simulink model "Simplus_1OL_2GFL"  (R2022b)
settings: Solver=ode3  StartTime=0.0  StopTime=35  FixedStep=Ts  RelTol=1e-3  EnableMultiTasking=on
InitFcn:
  | Ts = 100e-6;
model workspace (MAT data in the model file):
  Fbase = 50
  Filter_Ind = 0.00435
  Test_Interval = 5
  VDCref = 48
undefined symbols (not defined in the file): DiscIntNeverNeededParam
libraries: rtpi x45, spsabctodq0Lib x2, slpidlib x1, spsdq0toabcLib x1, simulink x1
settings Model: ModifiedByFormat=The MathWorks Inc.  SimulationMode=external  ExtModeTrigDuration=350000  ExtModeLogAll=off  Creator=The MathWorks, Inc.  LastModifiedBy=The MathWorks Inc.
settings SolverCC: AlgebraicLoopSolver=TrustRegion  PositivePriorityOrder=on  AutoInsertRateTranBlk=on
settings DataIOCC: LimitDataPoints=on  SaveFormat=Array  ReturnWorkspaceOutputs=off
settings OptimizationCC: EnhancedBackFolding=on  PassReuseOutputArgsThreshold=0  LocalBlockOutputs=off  EfficientMapNaN2IntZero=off  MaxStackSize=64  OptimizeBlockOrder=speed  DifferentSizesBufferReuse=on
settings DebuggingCC: UnderspecifiedInitializationDetection=Classic  MergeDetectMultiDrivingBlocksExec=none  SolverPrmCheckMsg=warning  ParameterTunabilityLossMsg=error  UnconnectedInputMsg=warning  UnconnectedOutputMsg=warning  UnconnectedLineMsg=warning  AllowSymbolicDim=off  SFUnexpectedBacktrackingDiag=warning  SFNoUnconditionalDefaultTransitionDiag=warning  SFExecutionAtInitializationDiag=none  SFMachineParentedDataDiag=warning  ArithmeticOperatorsInVariantConditions=warning
settings HardwareCC: ProdBitPerPointer=32  ProdBitPerSizeT=32  ProdBitPerPtrDiffT=32  ProdLargestAtomicInteger=Long  ProdLargestAtomicFloat=Double  ProdWordSize=32  ProdHWDeviceType=ARM Compatible->ARM Cortex  UseEmbeddedCoderFeatures=off
settings ModelReferenceCC: EnableRefExpFcnMdlSchedulingChecks=on  PropagateSignalLabelsOutOfModel=off
settings SFSimCC: SimUseLocalCustomCode=off  SimParseCustomCode=off  MATLABDynamicMemAlloc=off  CustomCodeUndefinedFunction=UseInterfaceOnly
settings RTWCC: Description=Simplus  SystemTargetFile=simplus.tlc  TemplateMakefile=simplex.tmf  RTWUseLocalCustomCode=off  RTWUseSimCustomCode=on  Toolchain=Simplus Xenomai ARM32  BuildConfiguration=Faster Runs
settings CodeAppCC: OperatorAnnotations=on  MangleLength=10  StateflowObjectComments=on
settings STFCustomTargetCC: TargetLangStandard=C99 (ISO)  GenerateFullHeader=off  ConcurrentExecutionCompliant=on  GRTInterface=on  UseToolchainInfoCompliant=on  SystemTargetFile=simplus.tlc
settings GRTTargetCC: GenerateFullHeader=off  ParMdlRefBuildCompliant=off  CompOptLevelCompliant=off  CombineOutputUpdateFcns=off  MatFileLogging=off  CPPClassGenCompliant=off  GRTInterface=on  ExtMode=on  ExtModeMexArgs='192.168.10.109', 0, 17725
settings ConfigComp: CovMetricSettings=dw  CovSaveCumulativeToWorkspaceVar=on  CovSaveSingleToWorkspaceVar=on  CovExternalEMLEnable=off  CovSFcnEnable=off

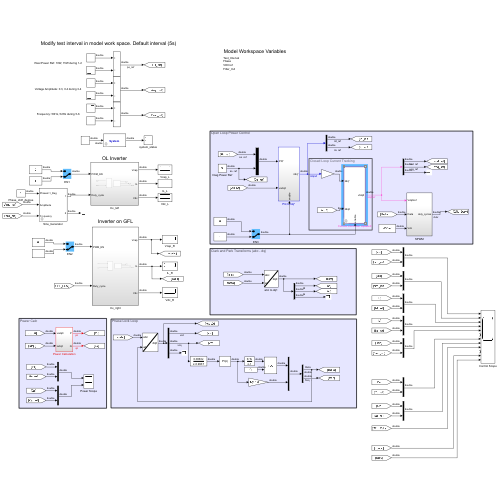
[thumbnail: Simulink's stored preview of the top-level diagram]
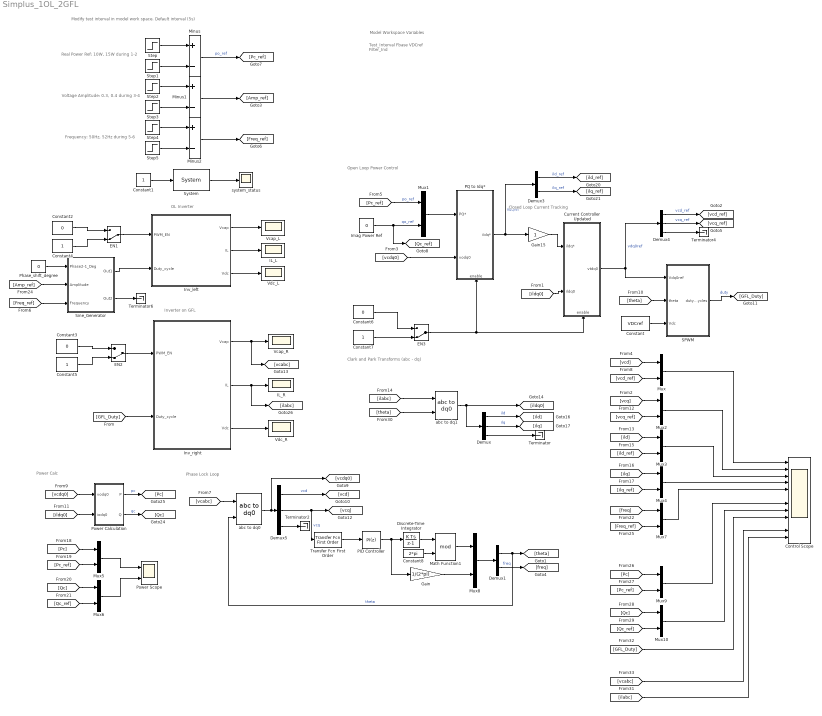
== system Simplus_1OL_2GFL ==
  note: Real Power Ref: 10W, 15W during 1-2
  note: Clark and Park Transforms (abc - dq)
  note: Closed Loop Current Tracking
  note: Phase Lock Loop
  note: Inverter on GFL
  note: Power Calc
  note: Open Loop Power Control
  note: OL Inverter
  note: Modify test interval in model work space. Default interval (5s)
  note: Voltage Amplitude: 0.3, 0.4 during 3-4
  note: Frequency: 50Hz, 52Hz during 5-6
  note: Test_Interval
      | Fbase
      | VDCref
      | Filter_Ind
  note: Model Workspace Variables
  Constant : Constant  Value=VDCref
  Constant{1,4..5,7} (4 alike) : Constant
  Constant2 : Constant  Value=0
  Constant3 : Constant  Value=0
  Constant6 : Constant  Value=0
  Constant8 : Constant  Value=2*pi
  Control Scope : Scope  NumInputPorts=12
  Current Controller Updated : Subsystem  mask{Id_Proportional=1.22, Id_Integral=957}
      mask prompts: Id_Proportional "Kp"; Id_Integral "Ki"
      settings: PortSchema="{\"entries\":[{\"content\":{\"sides\":[{\"content\":{\"connectorIds\":[\"In1\",\"In2\"]},\"type\":\"ConnectorPlacement.EquallySpacedRectSide\",\"uuid\":\"134caf41-c34b-48d0-a71a-522329c40d8c\"},{\"content\":{\"connectorIds\":[\"Out1\"],\"side\":\"RIGHT\"},\"type\":\"ConnectorPlacement.EquallySpacedRectSide\",\"uuid\":\"de6d8359-09d9-4cb7-8990-bc4b6d48f18d\"},{\"content\":{\"connectorIds\":[],\"side\":\"TOP\"},\"type\":\"ConnectorPlacement.EquallySpacedRectSide\",\"uuid\":\"e2785d07-2ead-4d42-94ac-8025f550e46a\"},{\"content\":{\"connectorIds\":[\"In3\"],\"side\":\"BOTTOM\"},\"type\":\"ConnectorPlacement.EquallySpacedRectSide\",\"uuid\":\"a912a274-012c-4cba-911c-beb79bb7dc91\"}]},\"type\":\"ConnectorPlacement.EquallySpacedConnector\",\"uuid\":\"3c498838-bb9a-4b09-bf48-00f71cabf7b4\"}],\"packageUris\":[\"http://schema.mathworks.com/mf0/Connector/R2020b\"],\"version\":\"1.0\"}"
  Demux : Demux  Outputs=3
  Demux1 : Demux  Outputs=2
  Demux3 : Demux  Outputs=2
  Demux4 : Demux  Outputs=3
  Demux5 : Demux  Outputs=3
  Discrete-Time Integrator : DiscreteIntegrator  SampleTime=Ts  ICPrevOutput=DiscIntNeverNeededParam  ICPrevScaledInput=DiscIntNeverNeededParam
  EN1 : ManualSwitch  CurrentSetting=0
  EN2 : ManualSwitch  CurrentSetting=0
  EN3 : ManualSwitch  CurrentSetting=0
  Gain : Gain  Gain=1/(2*pi)
  Gain15 : Gain
  IL_L : Scope
  IL_R : Scope
  Imag Power Ref : Constant  Value=0
  Inv_left : Subsystem
  Inv_right : Subsystem
  Math Function1 : Math  Operator=mod  SignedPower=on
  Minus : Sum  Inputs=+-
  Minus1 : Sum  Inputs=+-
  Minus2 : Sum  Inputs=+-
  Mux{,1..10} (11 alike) : Mux  Inputs=2
  PID Controller : slpidlib/PID Controller  Controller=PI  Form=Parallel  TimeDomain=Discrete-time  UseExternalTs=off  SampleTime=Ts  IntegratorMethod=Forward Euler  FilterMethod=Forward Euler  ControllerParametersSource=internal  P=2.4  I=1.52  UseKiTs=off  D=0  N=100  UseFilter=on  TunerSelectOption=Transfer Function Based (PID Tuner App)  InitialConditionSource=internal  InitialConditionForIntegrator=2*pi*Fbase  InitialConditionForFilter=0  DifferentiatorICPrevScaledInput=0  ExternalReset=none  TrackingMode=off  Kt=1  LimitOutput=off  SatLimitsSource=internal  UpperSaturationLimit=inf  LowerSaturationLimit=-inf  LinearizeAsGain=on  AntiWindupMode=none  Kb=1  LimitIntegrator=off  UpperIntegratorSaturationLimit=inf  LowerIntegratorSaturationLimit=-inf  POutMin=[]  POutMax=[]  IOutMin=[]  IOutMax=[]  DOutMin=[]  DOutMax=[]  NOutMin=[]  NOutMax=[]  SumOutMin=[]  SumOutMax=[]  SaturationOutMin=[]  SaturationOutMax=[]  PParamMin=[]  PParamMax=[]  IParamMin=[]  IParamMax=[]  DParamMin=[]  DParamMax=[]  NParamMin=[]  NParamMax=[]  KbParamMin=[]  KbParamMax=[]  KtParamMin=[]  KtParamMax=[]  KbOutMin=[]  KbOutMax=[]  KtOutMin=[]  KtOutMax=[]  IntegratorOutMin=[]  IntegratorOutMax=[]  FilterOutMin=[]  FilterOutMax=[]  SumI1OutMin=[]  SumI1OutMax=[]  SumI2OutMin=[]  SumI2OutMax=[]  SumI3OutMin=[]  SumI3OutMax=[]  SumI4OutMin=[]  SumI4OutMax=[]  SumDOutMin=[]  SumDOutMax=[]  DifferentiatorOutMin=[]  DifferentiatorOutMax=[]  FilterDiffOutCoefMin=[]  FilterDiffOutCoefMax=[]  ReciprocalOutMin=[]  ReciprocalOutMax=[]  SumDenOutMin=[]  SumDenOutMax=[]  SumNumOutMin=[]  SumNumOutMax=[]  DivideOutMin=[]  DivideOutMax=[]  UdiffTsProdOutMin=[]  UdiffTsProdOutMax=[]  NTsProdOutMin=[]  NTsProdOutMax=[]  UintegralTsProdOutMin=[]  UintegralTsProdOutMax=[]  UngainTsProdOutMin=[]  UngainTsProdOutMax=[]  ClampingZeroOutDataTypeStr=Inherit: Inherit via back propagation  ClampingZeroOutMin=[]  ClampingZeroOutMax=[]  FilterDenConstantOutDataTypeStr=Inherit: Inherit via back propagation  FilterDenConstantOutMin=[]  FilterDenConstantOutMax=[]  PCopyOutDataTypeStr=Inherit: Inherit via back propagation  PCopyOutMin=[]  PCopyOutMax=[]  NCopyOutDataTypeStr=Inherit: Inherit via back propagation  NCopyOutMin=[]  NCopyOutMax=[]  IntegratorContinuousStateAttributes=''  IntegratorStateMustResolveToSignalObject=off  IntegratorRTWStateStorageClass=Auto  FilterContinuousStateAttributes=''  FilterStateMustResolveToSignalObject=off  FilterRTWStateStorageClass=Auto  ParallelPVariant=InternalParameters  IdealPVariant=Disabled  IVariant=InternalParameters  DVariant=Disabled  IntegratorVariant=Discrete  SatVariant=Disabled  AWVariant=Passthrough  PCopyVariant=Disabled  TRVariant=Disabled  FdbkBlocksVariant=Forward  IdealPFdbkVariant=Disabled  SatFdbkVariant=Disabled  DerivativeFilterVariant=Disabled  NVariant=Disabled  NCopyVariant=Disabled_SignalSpec  FilterICVariant=Disabled  IntegratorICVariant=InternalICs  ExternalResetVariant=Disabled  TRSumVariant=Passthrough  SumFdbkVariant=Disabled  SumVariant=Sum_PI  TsampFilterVariant=InternalTs  TsampNgainVariant=Passthrough  TsampIntegralVariant=Passthrough  ExternalSaturationOutDataTypeStr=Inherit: Same as second input
  PQ to Idq* : Subsystem
      settings: PortSchema="{\"entries\":[{\"content\":{\"sides\":[{\"content\":{\"connectorIds\":[\"In1\",\"In2\"]},\"type\":\"ConnectorPlacement.EquallySpacedRectSide\",\"uuid\":\"5271b3ed-46a4-4113-9b69-458d23b85fa2\"},{\"content\":{\"connectorIds\":[\"Out1\"],\"side\":\"RIGHT\"},\"type\":\"ConnectorPlacement.EquallySpacedRectSide\",\"uuid\":\"00fb532b-4b50-4607-a5c4-cd74a5a5fc42\"},{\"content\":{\"connectorIds\":[],\"side\":\"TOP\"},\"type\":\"ConnectorPlacement.EquallySpacedRectSide\",\"uuid\":\"05671b8e-b1fa-45d3-a4a8-1640aa1af326\"},{\"content\":{\"connectorIds\":[\"In3\"],\"side\":\"BOTTOM\"},\"type\":\"ConnectorPlacement.EquallySpacedRectSide\",\"uuid\":\"cfa1ca65-6f63-4245-906b-c8bf76b96ed3\"}]},\"type\":\"ConnectorPlacement.EquallySpacedConnector\",\"uuid\":\"bf062c94-390f-4409-83d1-f8a32d59f496\"}],\"packageUris\":[\"http://schema.mathworks.com/mf0/Connector/R2020b\"],\"version\":\"1.0\"}"
  Phase_shift_degree : Constant  Value=0
  Power Calculation : Subsystem
  Power Scope : Scope  NumInputPorts=2
  SPWM : Subsystem
  Sine_Generator : Subsystem
  Step : Step  Time=Test_Interval*1  Before=10  After=15
  Step1 : Step  Time=Test_Interval*2  After=5
  Step2 : Step  Time=Test_Interval*3  Before=0.3  After=0.4
  Step3 : Step  Time=Test_Interval*4  After=0.1
  Step4 : Step  Time=Test_Interval*5  Before=50  After=52  SampleTime=0
  Step5 : Step  Time=Test_Interval*6  After=2
  System : rtpi/System  Priority=-100  finger_print=015482637925  sync=Synchronous Series  div=4  estop=NONE
      settings: SourceProductName=Simplus Real-Time
  Terminator{,2,4,6} (4 alike) : Terminator
  Transfer Fcn First Order : simulink/Discrete/Transfer Fcn First Order  PoleZ=0.9937  ICPrevOutput=0.0  DoSatur=off
  Vcap_L : Scope
  Vcap_R : Scope
  Vdc_L : Scope
  Vdc_R : Scope
  abc to dq0 : spsabctodq0Lib/abc to dq0  Alignment=90 degrees behind phase A axis
  abc to dq1 : spsabctodq0Lib/abc to dq0  Alignment=90 degrees behind phase A axis
  system_status : Scope
  wires:
  System/1 -> system_status/1
  Constant1/1 -> System/1
  Constant2/1 -> EN1/1
  Constant4/1 -> EN1/2
  Constant5/1 -> EN2/2
  Constant3/1 -> EN2/1
  Inv_left/1(Vcap) -> Vcap_L/1
  EN1/1 -> Inv_left/1(PWM_EN)
  Sine_Generator/1(Out1) -> Inv_left/2(Duty_cycle)
  Inv_left/2(IL) -> IL_L/1
  Inv_left/3(Vdc) -> Vdc_L/1
  Inv_right/1(Vcap) -> [vcabc], Vcap_R/1
  EN2/1 -> Inv_right/1(PWM_EN)
  Inv_right/2(IL) -> [ilabc], IL_R/1
  Inv_right/3(Vdc) -> Vdc_R/1
  Phase_shift_degree/1 -> Sine_Generator/1(Phase2-1_Deg)
  Demux4/2 -> [vcq_ref]  "vcq_ref"
  Demux/2 -> [ilq]  "ilq"
  Demux4/3 -> Terminator4/1
  Demux3/2 -> [ilq_ref]  "ilq_ref"
  Demux/3 -> Terminator/1
  PQ to Idq*/1(iIdq*) -> Gain15/1, Demux3/1  "ildqref"
  Current Controller Updated/1(vtdq0) -> SPWM/1(Vdq0ref), Demux4/1  "vdq0ref"
  [theta] -> SPWM/2(theta)
  SPWM/1(duty_cycles) -> [GFL_Duty]  "duty"
  Power Calculation/2(Q) -> [Qc]  "qc"
  Demux/1 -> [ild]  "ild"
  EN3/1 -> Current Controller Updated/3(enable), PQ to Idq*/3(enable)
  Power Calculation/1(P) -> [Pc]  "pc"
  Demux3/1 -> [ild_ref]  "ild_ref"
  [ildq0] -> Power Calculation/2(iodq0)
  Demux4/1 -> [vcd_ref]  "vcd_ref"
  [vcdq0] -> Power Calculation/1(vodq0)
  Constant/1 -> SPWM/3(Vdc)
  Gain15/1 -> Current Controller Updated/1(ildq*)
  Sine_Generator/2(Out2) -> Terminator6/1
  [GFL_Duty] -> Inv_right/2(Duty_cycle)
  Constant6/1 -> EN3/1
  Constant7/1 -> EN3/2
  [vcd_ref] -> Mux/2
  [vcd] -> Mux/1
  [vcq] -> Mux2/1
  [vcq_ref] -> Mux2/2
  [ild] -> Mux3/1
  [ild_ref] -> Mux3/2
  [ilq] -> Mux4/1
  [ilq_ref] -> Mux4/2
  Mux/1 -> Control Scope/1
  Mux2/1 -> Control Scope/2
  Mux3/1 -> Control Scope/3
  Mux4/1 -> Control Scope/4
  PID Controller/1 -> Gain/1, Discrete-Time Integrator/1
  Gain/1 -> Mux8/2
  Discrete-Time Integrator/1 -> Math Function1/1
  Constant8/1 -> Math Function1/2
  Demux1/2 -> [freq]  "freq"
  Demux1/1 -> abc to dq0/2, [theta]  "theta"
  Mux8/1 -> Demux1/1
  abc to dq0/1 -> [vcdq0], Demux5/1
  Demux5/1 -> [vcd]  "vcd"
  Demux5/3 -> Terminator2/1
  Demux5/2 -> Transfer Fcn First Order/1, [vcq]  "vcq"
  [vcabc] -> abc to dq0/1
  [theta] -> abc to dq1/2
  abc to dq1/1 -> [ildq0], Demux/1
  Mux6/1 -> Power Scope/2
  [Pc_ref] -> Mux5/2
  [Pc] -> Mux5/1
  [Qc_ref] -> Mux6/2
  [Qc] -> Mux6/1
  Mux5/1 -> Power Scope/1
  [Pc] -> Mux9/1
  [Qc] -> Mux10/1
  [Pc_ref] -> Mux9/2
  [Qc_ref] -> Mux10/2
  [ilabc] -> Control Scope/12
  Mux9/1 -> Control Scope/7
  [vcabc] -> Control Scope/11
  Mux10/1 -> Control Scope/8
  [GFL_Duty] -> Control Scope/9
  Mux1/1 -> PQ to Idq*/1(PQ*)
  Imag Power Ref/1 -> [Qc_ref], Mux1/2  "qo_ref"
  [Pc_ref] -> Mux1/1  "po_ref"
  [vcdq0] -> PQ to Idq*/2(vodq0)
  [ildq0] -> Current Controller Updated/2(ildq0)
  [ilabc] -> abc to dq1/1
  Step/1 -> Minus/1
  Step1/1 -> Minus/2
  Step2/1 -> Minus1/1
  Step3/1 -> Minus1/2
  Step4/1 -> Minus2/1
  Step5/1 -> Minus2/2
  Minus/1 -> [Pc_ref]  "po_ref"
  Minus1/1 -> [Amp_ref]
  Minus2/1 -> [Freq_ref]
  [Amp_ref] -> Sine_Generator/2(Amplitude)
  [Freq_ref] -> Sine_Generator/3(Frequency)
  [Freq_ref] -> Mux7/2
  [freq] -> Mux7/1
  Mux7/1 -> Control Scope/5
  Math Function1/1 -> Mux8/1
  Transfer Fcn First Order/1 -> PID Controller/1

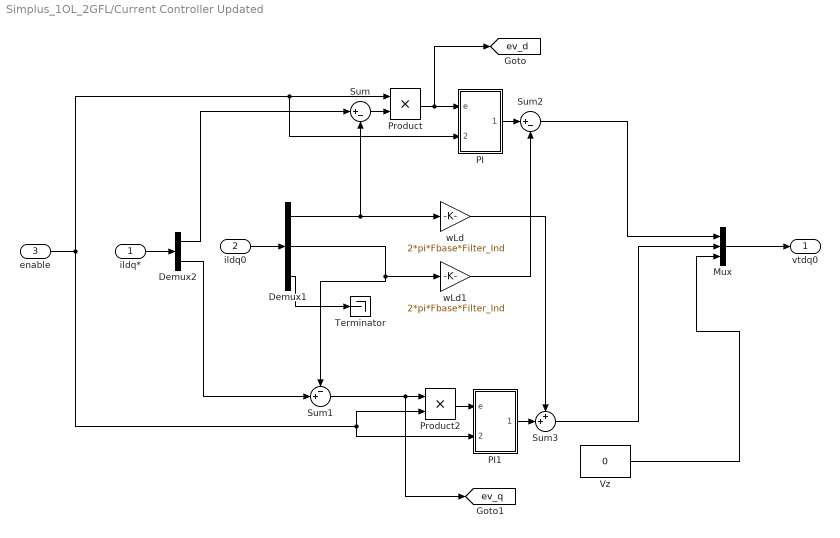
== system Simplus_1OL_2GFL/Current Controller Updated ==
  ildq* : Inport
  ildq0 : Inport  Port=2
  enable : Inport  Port=3
  Demux1 : Demux  Outputs=3
  Demux2 : Demux  Outputs=2
  Mux : Mux  Inputs=3
  PI : Subsystem
  PI1 : Subsystem
  Product : Product  RndMeth=Zero
  Product2 : Product  RndMeth=Zero
  Sum : Sum  Inputs=|+-
  Sum1 : Sum  Inputs=-+|
  Sum2 : Sum  Inputs=|+-
  Sum3 : Sum  Inputs=++|
  Terminator : Terminator
  Vz : Constant  Value=0
  wLd : Gain  Gain=2*pi*Fbase*Filter_Ind
  wLd1 : Gain  Gain=2*pi*Fbase*Filter_Ind
  vtdq0 : Outport
  tag scope: ev_d=global, ev_q=global
  wires:
  Sum2/1 -> Mux/1
  Sum3/1 -> Mux/2
  ildq0/1 -> Demux1/1
  Mux/1 -> vtdq0/1
  Demux1/3 -> Terminator/1
  ildq*/1 -> Demux2/1
  Demux2/1 -> Sum/1
  Demux2/2 -> Sum1/2
  Product/1 -> [ev_d], PI/1(e)
  Sum1/1 -> [ev_q], Product2/1
  PI/1(Out) -> Sum2/1
  wLd/1 -> Sum3/1
  wLd1/1 -> Sum2/2
  PI1/1(Out) -> Sum3/2
  Demux1/2 -> Sum1/1, wLd1/1
  Demux1/1 -> wLd/1, Sum/2
  Product2/1 -> PI1/1(e)
  Sum/1 -> Product/2
  enable/1 -> Product/1, PI/2(RST), PI1/2(RST), Product2/2
  Vz/1 -> Mux/3

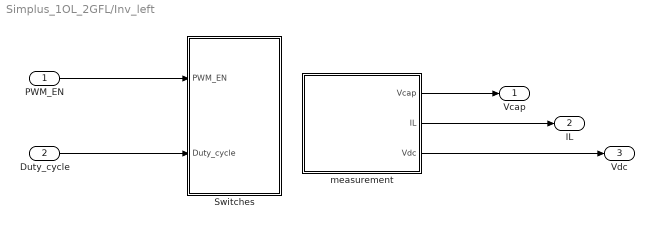
== system Simplus_1OL_2GFL/Inv_left ==
  PWM_EN : Inport
  Duty_cycle : Inport  Port=2
  Switches : Subsystem
  measurement : Subsystem
  Vcap : Outport
  IL : Outport  Port=2
  Vdc : Outport  Port=3
  wires:
  Duty_cycle/1 -> Switches/2(Duty_cycle)
  PWM_EN/1 -> Switches/1(PWM_EN)
  measurement/3(Vdc) -> Vdc/1
  measurement/2(IL) -> IL/1
  measurement/1(Vcap) -> Vcap/1

== system Simplus_1OL_2GFL/Inv_right ==
  PWM_EN : Inport
  Duty_cycle : Inport  Port=2
  Switches : Subsystem
  measurement : Subsystem
  Vcap : Outport
  IL : Outport  Port=2
  Vdc : Outport  Port=3
  wires:
  measurement/1(Vcap) -> Vcap/1
  measurement/2(IL) -> IL/1
  measurement/3(Vdc) -> Vdc/1
  PWM_EN/1 -> Switches/1(PWM_EN)
  Duty_cycle/1 -> Switches/2(Duty_cycle)

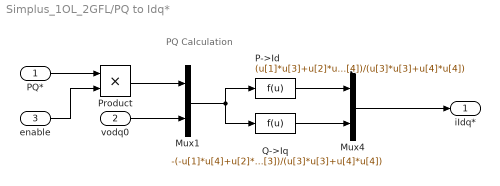
== system Simplus_1OL_2GFL/PQ to Idq* ==
  note: PQ Calculation
  PQ* : Inport
  vodq0 : Inport  Port=2
  enable : Inport  Port=3
  Mux1 : Mux  Inputs=2
  Mux4 : Mux  Inputs=2
  P->Id : Fcn  Expr=(u[1]*u[3]+u[2]*u[4])/(u[3]*u[3]+u[4]*u[4])
  Product : Product  RndMeth=Zero
  Q->Iq : Fcn  Expr=-(-u[1]*u[4]+u[2]*u[3])/(u[3]*u[3]+u[4]*u[4])
  iIdq* : Outport
  wires:
  enable/1 -> Product/2
  Product/1 -> Mux1/1
  Mux1/1 -> P->Id/1, Q->Iq/1
  P->Id/1 -> Mux4/1
  Q->Iq/1 -> Mux4/2
  Mux4/1 -> iIdq*/1
  vodq0/1 -> Mux1/2
  PQ*/1 -> Product/1

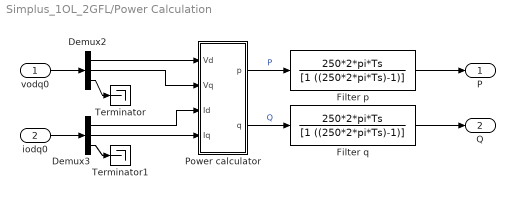
== system Simplus_1OL_2GFL/Power Calculation ==
  vodq0 : Inport
  iodq0 : Inport  Port=2
  Demux2 : Demux  Outputs=3
  Demux3 : Demux  Outputs=3
  Filter p : DiscreteTransferFcn  Numerator=250*2*pi*Ts  Denominator=[1 ((250*2*pi*Ts)-1)]  SampleTime=Ts
  Filter q : DiscreteTransferFcn  Numerator=250*2*pi*Ts  Denominator=[1 ((250*2*pi*Ts)-1)]  SampleTime=Ts
  Power calculator : Subsystem
  Terminator : Terminator
  Terminator1 : Terminator
  P : Outport
  Q : Outport  Port=2
  wires:
  vodq0/1 -> Demux2/1
  Demux2/1 -> Power calculator/1(Vd)
  Demux2/2 -> Power calculator/2(Vq)
  Demux3/1 -> Power calculator/3(Id)
  Demux3/2 -> Power calculator/4(Iq)
  iodq0/1 -> Demux3/1
  Power calculator/1(p) -> Filter p/1  "P"
  Power calculator/2(q) -> Filter q/1  "Q"
  Demux2/3 -> Terminator/1
  Demux3/3 -> Terminator1/1
  Filter p/1 -> P/1
  Filter q/1 -> Q/1

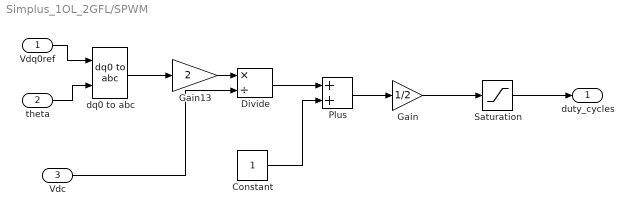
== system Simplus_1OL_2GFL/SPWM ==
  Vdq0ref : Inport
  theta : Inport  Port=2
  Vdc : Inport  Port=3
  Constant : Constant
  Divide : Product  Inputs=*/
  Gain : Gain  Gain=1/2
  Gain13 : Gain  Gain=2
  Plus : Sum
  Saturation : Saturate  UpperLimit=0.9  LowerLimit=0.1
  dq0 to abc : spsdq0toabcLib/dq0 to abc  Alignment=90 degrees behind phase A axis
  duty_cycles : Outport
  wires:
  Vdq0ref/1 -> dq0 to abc/1
  Gain/1 -> Saturation/1
  theta/1 -> dq0 to abc/2
  Constant/1 -> Plus/2
  Plus/1 -> Gain/1
  Saturation/1 -> duty_cycles/1
  dq0 to abc/1 -> Gain13/1
  Gain13/1 -> Divide/1
  Vdc/1 -> Divide/2
  Divide/1 -> Plus/1

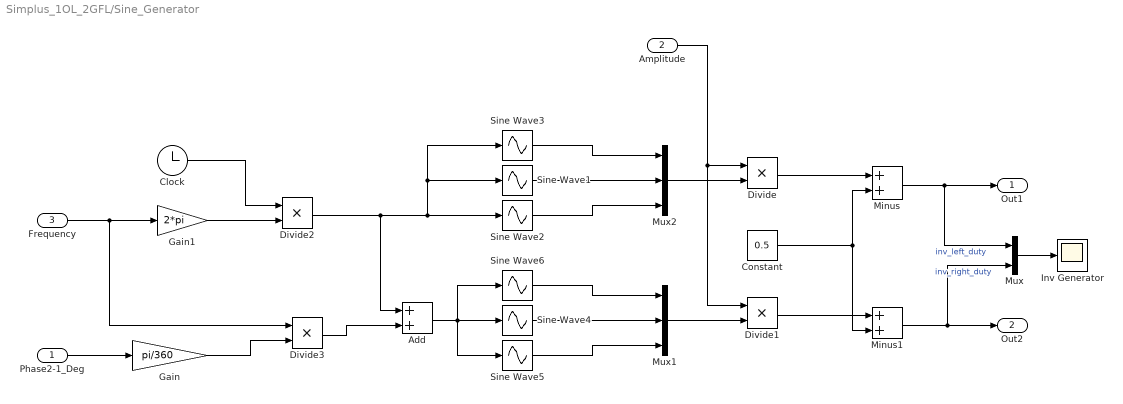
== system Simplus_1OL_2GFL/Sine_Generator ==
  Phase2-1_Deg : Inport
  Amplitude : Inport  Port=2
  Frequency : Inport  Port=3
  Add : Sum
  Clock : Clock
  Constant : Constant  Value=0.5
  Divide{,1..3} (4 alike) : Product  Inputs=**
  Gain : Gain  Gain=pi/360
  Gain1 : Gain  Gain=2*pi
  Inv Generator : Scope
  Minus : Sum
  Minus1 : Sum
  Mux : Mux  Inputs=2
  Mux1 : Mux  Inputs=3
  Mux2 : Mux  Inputs=3
  Sine Wave1 : Sin  TimeSource=Use external signal  Phase=-2*pi/3
  Sine Wave2 : Sin  TimeSource=Use external signal  Phase=2*pi/3
  Sine Wave3 : Sin  TimeSource=Use external signal
  Sine Wave4 : Sin  TimeSource=Use external signal  Phase=-2*pi/3
  Sine Wave5 : Sin  TimeSource=Use external signal  Phase=2*pi/3
  Sine Wave6 : Sin  TimeSource=Use external signal
  Out1 : Outport
  Out2 : Outport  Port=2
  wires:
  Add/1 -> Sine Wave6/1, Sine Wave5/1, Sine Wave4/1
  Sine Wave3/1 -> Mux2/1
  Divide2/1 -> Add/1, Sine Wave1/1, Sine Wave3/1, Sine Wave2/1
  Sine Wave6/1 -> Mux1/1
  Divide3/1 -> Add/2
  Sine Wave5/1 -> Mux1/3
  Sine Wave4/1 -> Mux1/2
  Sine Wave1/1 -> Mux2/2
  Sine Wave2/1 -> Mux2/3
  Minus/1 -> Out1/1, Mux/1  "inv_left_duty"
  Phase2-1_Deg/1 -> Gain/1
  Mux2/1 -> Divide/2
  Mux1/1 -> Divide1/2
  Amplitude/1 -> Divide/1, Divide1/1
  Gain1/1 -> Divide2/2
  Frequency/1 -> Divide3/1, Gain1/1
  Divide/1 -> Minus/1
  Divide1/1 -> Minus1/1
  Constant/1 -> Minus1/2, Minus/2
  Clock/1 -> Divide2/1
  Gain/1 -> Divide3/2
  Minus1/1 -> Out2/1, Mux/2  "inv_right_duty"
  Mux/1 -> Inv Generator/1

== system Simplus_1OL_2GFL/Current Controller Updated/PI ==
  e : Inport
  RST : Inport  Port=2
  Discrete-Time Integrator : DiscreteIntegrator  gainval=1  ExternalReset=either  SampleTime=Ts  LimitOutput=on  UpperSaturationLimit=20000  LowerSaturationLimit=-20000  ICPrevOutput=DiscIntNeverNeededParam  ICPrevScaledInput=DiscIntNeverNeededParam
  Ki : Gain  Gain=Id_Integral  SaturateOnIntegerOverflow=on  OutDataTypeStr=Inherit: Same as input  ParamDataTypeStr=Inherit: Same as input
  Kp : Gain  Gain=Id_Proportional  SaturateOnIntegerOverflow=on  OutDataTypeStr=Inherit: Same as input  ParamDataTypeStr=Inherit: Same as input
  Sum4 : Sum  SaturateOnIntegerOverflow=on
  Out : Outport
  wires:
  Ki/1 -> Discrete-Time Integrator/1
  Kp/1 -> Sum4/1
  e/1 -> Ki/1, Kp/1
  Discrete-Time Integrator/1 -> Sum4/2
  Sum4/1 -> Out/1
  RST/1 -> Discrete-Time Integrator/2

== system Simplus_1OL_2GFL/Current Controller Updated/PI1 ==
  e : Inport
  RST : Inport  Port=2
  Discrete-Time Integrator : DiscreteIntegrator  gainval=1  ExternalReset=either  SampleTime=Ts  LimitOutput=on  UpperSaturationLimit=20000  LowerSaturationLimit=-20000  ICPrevOutput=DiscIntNeverNeededParam  ICPrevScaledInput=DiscIntNeverNeededParam
  Ki : Gain  Gain=Id_Integral  SaturateOnIntegerOverflow=on  OutDataTypeStr=Inherit: Same as input  ParamDataTypeStr=Inherit: Same as input
  Kp : Gain  Gain=Id_Proportional  SaturateOnIntegerOverflow=on  OutDataTypeStr=Inherit: Same as input  ParamDataTypeStr=Inherit: Same as input
  Sum4 : Sum  SaturateOnIntegerOverflow=on
  Out : Outport
  wires:
  Ki/1 -> Discrete-Time Integrator/1
  Kp/1 -> Sum4/1
  e/1 -> Ki/1, Kp/1
  Discrete-Time Integrator/1 -> Sum4/2
  Sum4/1 -> Out/1
  RST/1 -> Discrete-Time Integrator/2

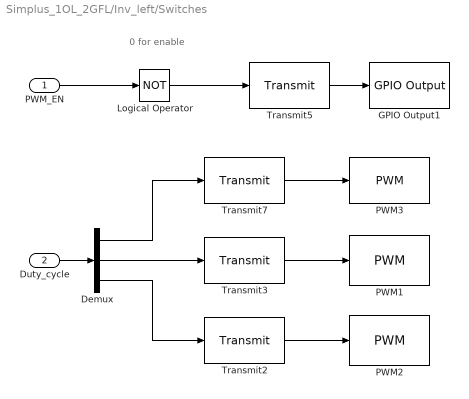
== system Simplus_1OL_2GFL/Inv_left/Switches ==
  note: 0 for enable
  PWM_EN : Inport
  Duty_cycle : Inport  Port=2
  Demux : Demux  Outputs=3
  GPIO Output1 : rtpi/GPIO Output  finger_print=115482637925  blk_num=1  gpio_num=1  gpio1=18  od1=off  gpio2=0  od2=off  gpio3=0  od3=off  gpio4=0  od4=off  gpio5=0  od5=off  gpio6=0  od6=off  gpio7=0  od7=off  gpio8=0  od8=off  gpio9=0  od9=off  gpio10=0  od10=off  gpio11=0  od11=off  gpio12=0  od12=off  gpio13=0  od13=off  gpio14=0  od14=off  gpio15=0  od15=off  gpio16=0  od16=off  dir=1
      settings: SourceProductName=Simplus Real-Time
  Logical Operator : Logic  Operator=NOT  AllPortsSameDT=off  OutDataTypeStr=boolean
  PWM1 : rtpi/PWM  finger_print=115482637925  blk_num=1  pwmx=5  sync=on  mode=Normal  input=Duty Cycle  data_type=float  trigger_a=Zero  trigger_b=Zero  clock=1  tdead=2  period=10000  duty=0.5  phase=0.0
      settings: SourceProductName=Simplus Real-Time
  PWM2 : rtpi/PWM  finger_print=115482637925  blk_num=2  pwmx=6  sync=on  mode=Normal  input=Duty Cycle  data_type=float  trigger_a=Zero  trigger_b=Zero  clock=1  tdead=2  period=10000  duty=0.5  phase=0.0
      settings: SourceProductName=Simplus Real-Time
  PWM3 : rtpi/PWM  finger_print=115482637925  blk_num=3  pwmx=4  sync=on  mode=Normal  input=Duty Cycle  data_type=float  trigger_a=Zero  trigger_b=Zero  clock=1  tdead=2  period=10000  duty=0.5  phase=0.0
      settings: SourceProductName=Simplus Real-Time
  Transmit2 : rtpi/Transmit  Priority=10  finger_print=115482637925  blk_num=1  data_type=4  conv_type=single
      settings: SourceProductName=Simplus Real-Time
  Transmit3 : rtpi/Transmit  Priority=10  finger_print=115482637925  blk_num=2  data_type=4  conv_type=single
      settings: SourceProductName=Simplus Real-Time
  Transmit5 : rtpi/Transmit  finger_print=115482637925  blk_num=3  data_type=2  conv_type=uint16
      settings: SourceProductName=Simplus Real-Time
  Transmit7 : rtpi/Transmit  Priority=10  finger_print=115482637925  blk_num=4  data_type=4  conv_type=single
      settings: SourceProductName=Simplus Real-Time
  wires:
  Transmit2/1 -> PWM2/1
  Transmit3/1 -> PWM1/1
  Transmit7/1 -> PWM3/1
  Duty_cycle/1 -> Demux/1
  Demux/2 -> Transmit3/1
  Demux/1 -> Transmit7/1
  Demux/3 -> Transmit2/1
  Transmit5/1 -> GPIO Output1/1
  Logical Operator/1 -> Transmit5/1
  PWM_EN/1 -> Logical Operator/1

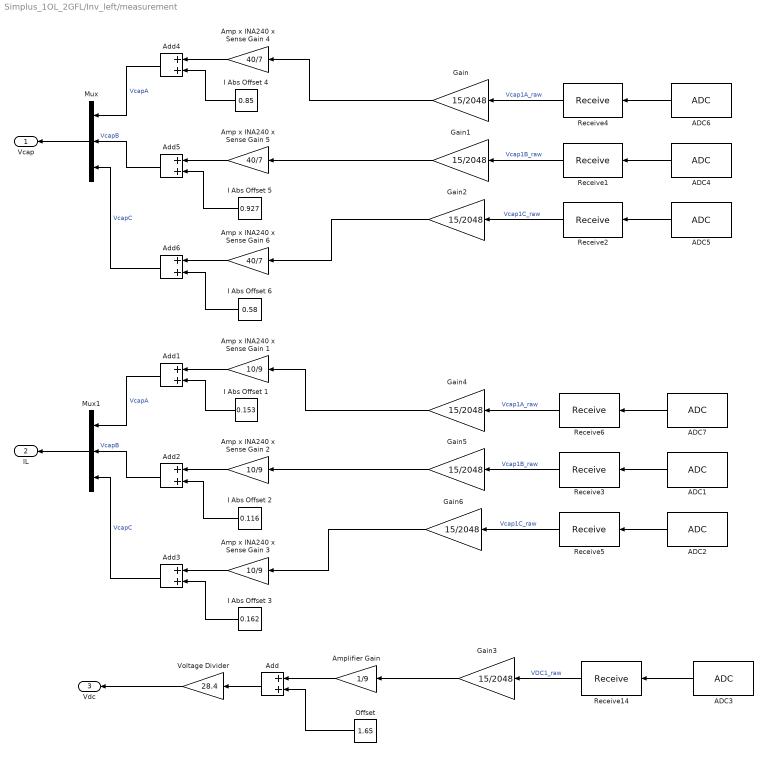
== system Simplus_1OL_2GFL/Inv_left/measurement ==
  ADC1 : rtpi/ADC  finger_print=115482637925  blk_num=1  adcx=D  prior=2  pin=D2  trigger=PWM4A  data_type=int16  gain=1  rsrc=100  offset=AC  protect=Enabled  max=1500  min=-1500
      settings: SourceProductName=Simplus Real-Time
  ADC2 : rtpi/ADC  finger_print=115482637925  blk_num=2  adcx=D  prior=3  pin=D3  trigger=PWM4A  data_type=int16  gain=1  rsrc=100  offset=AC  protect=Enabled  max=1500  min=-1500
      settings: SourceProductName=Simplus Real-Time
  ADC3 : rtpi/ADC  finger_print=115482637925  blk_num=3  adcx=D  prior=4  pin=D4  trigger=PWM4A  data_type=int16  gain=1  rsrc=100  offset=AC  protect=Enabled  max=1500  min=-2048
      settings: SourceProductName=Simplus Real-Time
  ADC4 : rtpi/ADC  finger_print=115482637925  blk_num=4  adcx=C  prior=2  pin=C2  trigger=PWM4A  data_type=int16  gain=1  rsrc=100  offset=AC  protect=Enabled  max=1500  min=-1500
      settings: SourceProductName=Simplus Real-Time
  ADC5 : rtpi/ADC  finger_print=115482637925  blk_num=5  adcx=C  prior=3  pin=C3  trigger=PWM4A  data_type=int16  gain=1  rsrc=100  offset=AC  protect=Enabled  max=1500  min=-1500
      settings: SourceProductName=Simplus Real-Time
  ADC6 : rtpi/ADC  finger_print=115482637925  blk_num=6  adcx=C  prior=1  pin=C1  trigger=PWM4A  data_type=int16  gain=1  rsrc=100  offset=AC  protect=Enabled  max=1500  min=-1500
      settings: SourceProductName=Simplus Real-Time
  ADC7 : rtpi/ADC  finger_print=115482637925  blk_num=7  adcx=D  prior=1  pin=D1  trigger=PWM4A  data_type=int16  gain=1  rsrc=100  offset=AC  protect=Enabled  max=1500  min=-1500
      settings: SourceProductName=Simplus Real-Time
  Add{,1..6} (7 alike) : Sum
  Amp x INA240 x Sense Gain 1 : Gain  Gain=10/9
  Amp x INA240 x Sense Gain 2 : Gain  Gain=10/9
  Amp x INA240 x Sense Gain 3 : Gain  Gain=10/9
  Amp x INA240 x Sense Gain 4 : Gain  Gain=40/7
  Amp x INA240 x Sense Gain 5 : Gain  Gain=40/7
  Amp x INA240 x Sense Gain 6 : Gain  Gain=40/7
  Amplifier Gain : Gain  Gain=1/9
  Gain{,1..6} (7 alike) : Gain  Gain=15/2048
  I Abs Offset 1 : Constant  Value=0.153
  I Abs Offset 2 : Constant  Value=0.116
  I Abs Offset 3 : Constant  Value=0.162
  I Abs Offset 4 : Constant  Value=0.85
  I Abs Offset 5 : Constant  Value=0.927
  I Abs Offset 6 : Constant  Value=0.58
  Mux : Mux  Inputs=3
  Mux1 : Mux  Inputs=3
  Offset : Constant  Value=1.65
  Receive1 : rtpi/Receive  Priority=12  finger_print=115482637925  blk_num=1  data_type=2
      settings: SourceProductName=Simplus Real-Time
  Receive14 : rtpi/Receive  Priority=12  finger_print=115482637925  blk_num=2  data_type=2
      settings: SourceProductName=Simplus Real-Time
  Receive2 : rtpi/Receive  Priority=12  finger_print=115482637925  blk_num=3  data_type=2
      settings: SourceProductName=Simplus Real-Time
  Receive3 : rtpi/Receive  Priority=12  finger_print=115482637925  blk_num=4  data_type=2
      settings: SourceProductName=Simplus Real-Time
  Receive4 : rtpi/Receive  Priority=12  finger_print=115482637925  blk_num=5  data_type=2
      settings: SourceProductName=Simplus Real-Time
  Receive5 : rtpi/Receive  Priority=12  finger_print=115482637925  blk_num=6  data_type=2
      settings: SourceProductName=Simplus Real-Time
  Receive6 : rtpi/Receive  Priority=12  finger_print=115482637925  blk_num=7  data_type=2
      settings: SourceProductName=Simplus Real-Time
  Voltage Divider : Gain  Gain=28.4
  Vcap : Outport
  IL : Outport  Port=2
  Vdc : Outport  Port=3
  wires:
  ADC6/1 -> Receive4/1
  Receive4/1 -> Gain/1  "Vcap1A_raw"
  Amp x INA240 x Sense Gain 6/1 -> Add6/1
  I Abs Offset 6/1 -> Add6/2
  I Abs Offset 4/1 -> Add4/2
  Amp x INA240 x Sense Gain 4/1 -> Add4/1
  ADC5/1 -> Receive2/1
  Amp x INA240 x Sense Gain 5/1 -> Add5/1
  Receive1/1 -> Gain1/1  "Vcap1B_raw"
  I Abs Offset 5/1 -> Add5/2
  Receive2/1 -> Gain2/1  "Vcap1C_raw"
  ADC4/1 -> Receive1/1
  Amp x INA240 x Sense Gain 3/1 -> Add3/1
  Amp x INA240 x Sense Gain 1/1 -> Add1/1
  I Abs Offset 1/1 -> Add1/2
  Amp x INA240 x Sense Gain 2/1 -> Add2/1
  I Abs Offset 2/1 -> Add2/2
  I Abs Offset 3/1 -> Add3/2
  Receive14/1 -> Gain3/1  "VDC1_raw"
  ADC3/1 -> Receive14/1
  Add/1 -> Voltage Divider/1
  Amplifier Gain/1 -> Add/1
  Offset/1 -> Add/2
  Voltage Divider/1 -> Vdc/1
  Gain/1 -> Amp x INA240 x Sense Gain 4/1
  Gain1/1 -> Amp x INA240 x Sense Gain 5/1
  Gain2/1 -> Amp x INA240 x Sense Gain 6/1
  Gain3/1 -> Amplifier Gain/1
  Add4/1 -> Mux/1  "VcapA"
  Add5/1 -> Mux/2  "VcapB"
  Add6/1 -> Mux/3  "VcapC"
  Mux/1 -> Vcap/1
  ADC7/1 -> Receive6/1
  Gain4/1 -> Amp x INA240 x Sense Gain 1/1
  Gain5/1 -> Amp x INA240 x Sense Gain 2/1
  ADC1/1 -> Receive3/1
  ADC2/1 -> Receive5/1
  Receive3/1 -> Gain5/1  "Vcap1B_raw"
  Receive5/1 -> Gain6/1  "Vcap1C_raw"
  Gain6/1 -> Amp x INA240 x Sense Gain 3/1
  Receive6/1 -> Gain4/1  "Vcap1A_raw"
  Add3/1 -> Mux1/3  "VcapC"
  Mux1/1 -> IL/1
  Add1/1 -> Mux1/1  "VcapA"
  Add2/1 -> Mux1/2  "VcapB"

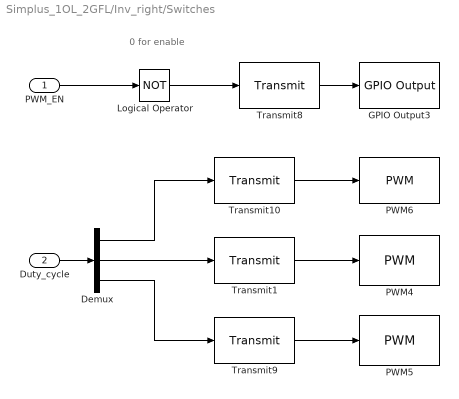
== system Simplus_1OL_2GFL/Inv_right/Switches ==
  note: 0 for enable
  PWM_EN : Inport
  Duty_cycle : Inport  Port=2
  Demux : Demux  Outputs=3
  GPIO Output3 : rtpi/GPIO Output  finger_print=115482637925  blk_num=2  gpio_num=1  gpio1=24  od1=off  gpio2=0  od2=off  gpio3=0  od3=off  gpio4=0  od4=off  gpio5=0  od5=off  gpio6=0  od6=off  gpio7=0  od7=off  gpio8=0  od8=off  gpio9=0  od9=off  gpio10=0  od10=off  gpio11=0  od11=off  gpio12=0  od12=off  gpio13=0  od13=off  gpio14=0  od14=off  gpio15=0  od15=off  gpio16=0  od16=off  dir=1
      settings: SourceProductName=Simplus Real-Time
  Logical Operator : Logic  Operator=NOT  AllPortsSameDT=off  OutDataTypeStr=boolean
  PWM4 : rtpi/PWM  finger_print=115482637925  blk_num=4  pwmx=2  sync=on  mode=Normal  input=Duty Cycle  data_type=float  trigger_a=Zero  trigger_b=Zero  clock=1  tdead=2  period=10000  duty=0.5  phase=0.0
      settings: SourceProductName=Simplus Real-Time
  PWM5 : rtpi/PWM  finger_print=115482637925  blk_num=5  pwmx=3  sync=on  mode=Normal  input=Duty Cycle  data_type=float  trigger_a=Zero  trigger_b=Zero  clock=1  tdead=2  period=10000  duty=0.5  phase=0.0
      settings: SourceProductName=Simplus Real-Time
  PWM6 : rtpi/PWM  finger_print=115482637925  blk_num=6  pwmx=1  sync=on  mode=Normal  input=Duty Cycle  data_type=float  trigger_a=Zero  trigger_b=Zero  clock=1  tdead=2  period=10000  duty=0.5  phase=0.0
      settings: SourceProductName=Simplus Real-Time
  Transmit1 : rtpi/Transmit  Priority=10  finger_print=115482637925  blk_num=5  data_type=4  conv_type=single
      settings: SourceProductName=Simplus Real-Time
  Transmit10 : rtpi/Transmit  Priority=10  finger_print=115482637925  blk_num=6  data_type=4  conv_type=single
      settings: SourceProductName=Simplus Real-Time
  Transmit8 : rtpi/Transmit  finger_print=115482637925  blk_num=7  data_type=2  conv_type=uint16
      settings: SourceProductName=Simplus Real-Time
  Transmit9 : rtpi/Transmit  Priority=10  finger_print=115482637925  blk_num=8  data_type=4  conv_type=single
      settings: SourceProductName=Simplus Real-Time
  wires:
  Duty_cycle/1 -> Demux/1
  PWM_EN/1 -> Logical Operator/1
  Demux/3 -> Transmit9/1
  Demux/1 -> Transmit10/1
  Demux/2 -> Transmit1/1
  Transmit9/1 -> PWM5/1
  Transmit1/1 -> PWM4/1
  Transmit10/1 -> PWM6/1
  Transmit8/1 -> GPIO Output3/1
  Logical Operator/1 -> Transmit8/1

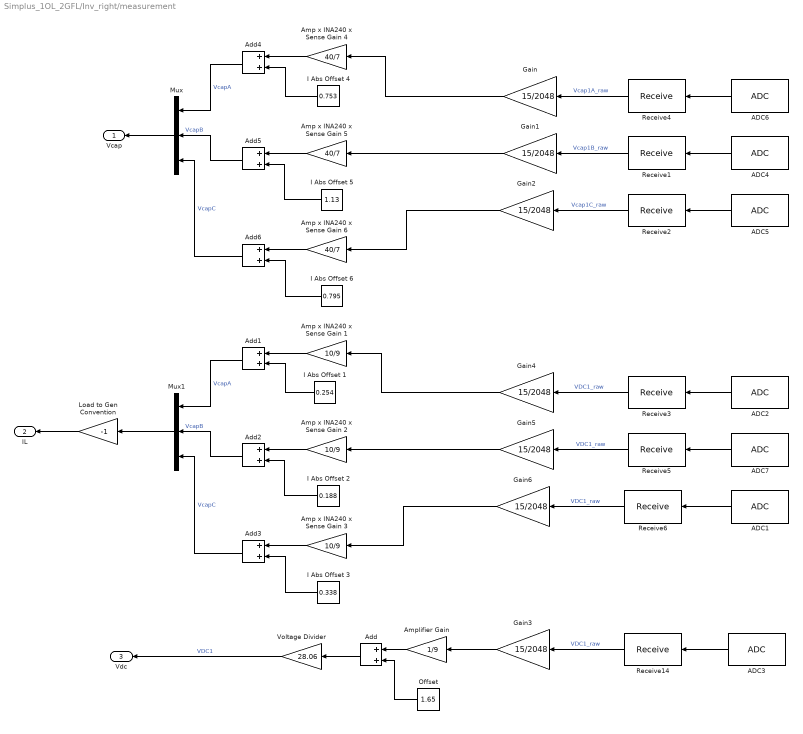
== system Simplus_1OL_2GFL/Inv_right/measurement ==
  ADC1 : rtpi/ADC  finger_print=115482637925  blk_num=8  adcx=A  prior=1  pin=A1  trigger=PWM1A  data_type=int16  gain=1  rsrc=100  offset=AC  protect=Enabled  max=1500  min=-1500
      settings: SourceProductName=Simplus Real-Time
  ADC2 : rtpi/ADC  finger_print=115482637925  blk_num=9  adcx=A  prior=2  pin=A2  trigger=PWM1A  data_type=int16  gain=1  rsrc=100  offset=AC  protect=Enabled  max=1500  min=-1500
      settings: SourceProductName=Simplus Real-Time
  ADC3 : rtpi/ADC  finger_print=115482637925  blk_num=10  adcx=A  prior=4  pin=A4  trigger=PWM1A  data_type=int16  gain=1  rsrc=100  offset=AC  protect=Enabled  max=1500  min=-2048
      settings: SourceProductName=Simplus Real-Time
  ADC4 : rtpi/ADC  finger_print=115482637925  blk_num=11  adcx=B  prior=2  pin=B3  trigger=PWM1A  data_type=int16  gain=1  rsrc=100  offset=AC  protect=Enabled  max=1500  min=-1500
      settings: SourceProductName=Simplus Real-Time
  ADC5 : rtpi/ADC  finger_print=115482637925  blk_num=12  adcx=B  prior=3  pin=B4  trigger=PWM1A  data_type=int16  gain=1  rsrc=100  offset=AC  protect=Enabled  max=1500  min=-1500
      settings: SourceProductName=Simplus Real-Time
  ADC6 : rtpi/ADC  finger_print=115482637925  blk_num=13  adcx=B  prior=1  pin=B2  trigger=PWM1A  data_type=int16  gain=1  rsrc=100  offset=AC  protect=Enabled  max=1500  min=-1500
      settings: SourceProductName=Simplus Real-Time
  ADC7 : rtpi/ADC  finger_print=115482637925  blk_num=14  adcx=A  prior=3  pin=A3  trigger=PWM1A  data_type=int16  gain=1  rsrc=100  offset=AC  protect=Enabled  max=1500  min=-1500
      settings: SourceProductName=Simplus Real-Time
  Add{,1..6} (7 alike) : Sum
  Amp x INA240 x Sense Gain 1 : Gain  Gain=10/9
  Amp x INA240 x Sense Gain 2 : Gain  Gain=10/9
  Amp x INA240 x Sense Gain 3 : Gain  Gain=10/9
  Amp x INA240 x Sense Gain 4 : Gain  Gain=40/7
  Amp x INA240 x Sense Gain 5 : Gain  Gain=40/7
  Amp x INA240 x Sense Gain 6 : Gain  Gain=40/7
  Amplifier Gain : Gain  Gain=1/9
  Gain{,1..6} (7 alike) : Gain  Gain=15/2048
  I Abs Offset 1 : Constant  Value=0.254
  I Abs Offset 2 : Constant  Value=0.188
  I Abs Offset 3 : Constant  Value=0.338
  I Abs Offset 4 : Constant  Value=0.753
  I Abs Offset 5 : Constant  Value=1.13
  I Abs Offset 6 : Constant  Value=0.795
  Load to Gen Convention : Gain  Gain=-1
  Mux : Mux  Inputs=3
  Mux1 : Mux  Inputs=3
  Offset : Constant  Value=1.65
  Receive1 : rtpi/Receive  Priority=12  finger_print=115482637925  blk_num=8  data_type=2
      settings: SourceProductName=Simplus Real-Time
  Receive14 : rtpi/Receive  Priority=12  finger_print=115482637925  blk_num=9  data_type=2
      settings: SourceProductName=Simplus Real-Time
  Receive2 : rtpi/Receive  Priority=12  finger_print=115482637925  blk_num=10  data_type=2
      settings: SourceProductName=Simplus Real-Time
  Receive3 : rtpi/Receive  Priority=12  finger_print=115482637925  blk_num=11  data_type=2
      settings: SourceProductName=Simplus Real-Time
  Receive4 : rtpi/Receive  Priority=12  finger_print=115482637925  blk_num=12  data_type=2
      settings: SourceProductName=Simplus Real-Time
  Receive5 : rtpi/Receive  Priority=12  finger_print=115482637925  blk_num=13  data_type=2
      settings: SourceProductName=Simplus Real-Time
  Receive6 : rtpi/Receive  Priority=12  finger_print=115482637925  blk_num=14  data_type=2
      settings: SourceProductName=Simplus Real-Time
  Voltage Divider : Gain  Gain=28.06
  Vcap : Outport
  IL : Outport  Port=2
  Vdc : Outport  Port=3
  wires:
  ADC6/1 -> Receive4/1
  Receive4/1 -> Gain/1  "Vcap1A_raw"
  Amp x INA240 x Sense Gain 6/1 -> Add6/1
  I Abs Offset 6/1 -> Add6/2
  I Abs Offset 4/1 -> Add4/2
  Amp x INA240 x Sense Gain 4/1 -> Add4/1
  ADC5/1 -> Receive2/1
  Amp x INA240 x Sense Gain 5/1 -> Add5/1
  Receive1/1 -> Gain1/1  "Vcap1B_raw"
  I Abs Offset 5/1 -> Add5/2
  Receive2/1 -> Gain2/1  "Vcap1C_raw"
  ADC4/1 -> Receive1/1
  Amp x INA240 x Sense Gain 3/1 -> Add3/1
  Amp x INA240 x Sense Gain 1/1 -> Add1/1
  I Abs Offset 1/1 -> Add1/2
  Amp x INA240 x Sense Gain 2/1 -> Add2/1
  I Abs Offset 2/1 -> Add2/2
  I Abs Offset 3/1 -> Add3/2
  Receive14/1 -> Gain3/1  "VDC1_raw"
  ADC3/1 -> Receive14/1
  Add/1 -> Voltage Divider/1
  Voltage Divider/1 -> Vdc/1  "VDC1"
  Amplifier Gain/1 -> Add/1
  Offset/1 -> Add/2
  Gain/1 -> Amp x INA240 x Sense Gain 4/1
  Gain1/1 -> Amp x INA240 x Sense Gain 5/1
  Gain2/1 -> Amp x INA240 x Sense Gain 6/1
  Gain3/1 -> Amplifier Gain/1
  Add4/1 -> Mux/1  "VcapA"
  Add5/1 -> Mux/2  "VcapB"
  Add6/1 -> Mux/3  "VcapC"
  Mux/1 -> Vcap/1
  Gain4/1 -> Amp x INA240 x Sense Gain 1/1
  Gain5/1 -> Amp x INA240 x Sense Gain 2/1
  Gain6/1 -> Amp x INA240 x Sense Gain 3/1
  Add3/1 -> Mux1/3  "VcapC"
  Mux1/1 -> Load to Gen Convention/1
  Add1/1 -> Mux1/1  "VcapA"
  Add2/1 -> Mux1/2  "VcapB"
  Receive3/1 -> Gain4/1  "VDC1_raw"
  ADC2/1 -> Receive3/1
  Receive5/1 -> Gain5/1  "VDC1_raw"
  ADC7/1 -> Receive5/1
  Receive6/1 -> Gain6/1  "VDC1_raw"
  ADC1/1 -> Receive6/1
  Load to Gen Convention/1 -> IL/1

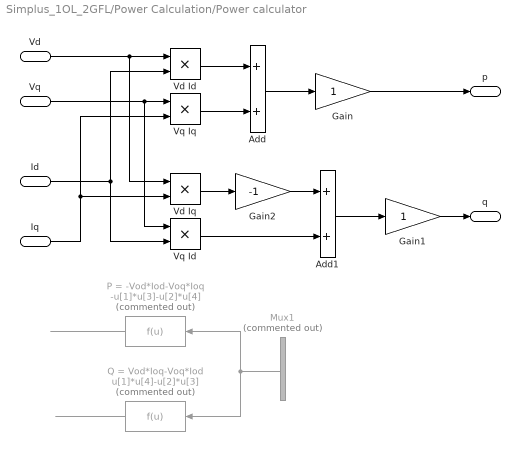
== system Simplus_1OL_2GFL/Power Calculation/Power calculator ==
  Vd : Inport
  Vq : Inport  Port=2
  Id : Inport  Port=3
  Iq : Inport  Port=4
  Add : Sum
  Add1 : Sum
  Gain : Gain
  Gain1 : Gain
  Gain2 : Gain  Gain=-1
  Mux1 : Mux  Commented=on
  P = -Vod*Iod-Voq*Ioq : Fcn  Commented=on  Expr=-u[1]*u[3]-u[2]*u[4]
  Q = Vod*Ioq-Voq*Iod : Fcn  Commented=on  Expr=u[1]*u[4]-u[2]*u[3]
  Vd Id : Product
  Vd Iq : Product
  Vq Id : Product
  Vq Iq : Product
  p : Outport
  q : Outport  Port=2
  wires:
  Q = Vod*Ioq-Voq*Iod/1 -> ?
  P = -Vod*Iod-Voq*Ioq/1 -> ?
  Mux1/1 -> Q = Vod*Ioq-Voq*Iod/1, P = -Vod*Iod-Voq*Ioq/1
  Gain/1 -> p/1
  Add/1 -> Gain/1
  Add1/1 -> Gain1/1
  Gain1/1 -> q/1
  Vd Id/1 -> Add/1
  Vq Iq/1 -> Add/2
  Vq Id/1 -> Add1/2
  Vd Iq/1 -> Gain2/1
  Vd/1 -> Vd Iq/1, Vd Id/1
  Id/1 -> Vd Id/2, Vq Id/2
  Vq/1 -> Vq Id/1, Vq Iq/1
  Iq/1 -> Vd Iq/2, Vq Iq/2
  Gain2/1 -> Add1/1
